simulink library "Fixed_Surface"  (Simulink 8.2)
settings: Solver=ode45  StartTime=0.0  StopTime=10.0  RelTol=1e-3
settings Model: Creator=lena.frank  LastModifiedBy=drhf

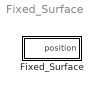
== system Fixed_Surface ==
  Fixed_Surface : Subsystem  mask(fixed surface){colangle=30, colazi=0, colrot=0}
      mask prompts: colangle "collector slope (0° = horizontal) [degree]"; colazi "collector azimuth (0° = south, -90° = east) [degree]"; colrot "collector rotation angle [degree]"
      mask help:
      | Set collector or surface to a fixed position.
      | All angles in degrees.
      mask init:
      | colangle = min(180, max(-180, colangle));
      | colazi = min(180, max(-180, colazi));
      | colrot = min(180, max(-180, colrot));
      mask Help: web(fullfile(path_carnot('help'),'Fixed_Surface.html'),'-helpbrowser')

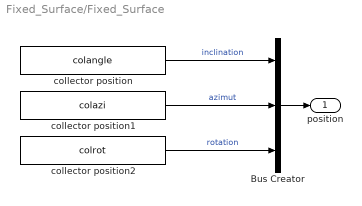
== system Fixed_Surface/Fixed_Surface ==
  Bus Creator : BusCreator  Inputs=3
  collector position : Constant  Value=colangle
  collector position1 : Constant  Value=colazi
  collector position2 : Constant  Value=colrot
  position : Outport
  wires:
  Bus Creator/1 -> position/1
  collector position/1 -> Bus Creator/1  "inclination"
  collector position1/1 -> Bus Creator/2  "azimut"
  collector position2/1 -> Bus Creator/3  "rotation"
